simulink model "reverb"  (R2024a)
settings: Solver=VariableStepAuto  StartTime=0.0  StopTime=1  RelTol=1e-3
model workspace (MAT data in the model file):
  Sig = Simulink.Signal
  Sig.DataType = 'auto'
  Sig.Dimensions = -1
  Sig.DimensionsMode = 'auto'
  Sig.Complexity = 'auto'
  Sig.SampleTime = -1
  Sig.SamplingMode = 'auto'
undefined symbols (not defined in the file or in its folder): DELAY, DELAY_DIFF, DIFF_GAIN, GAIN, MIX
libraries: dspvision x1
settings Model: Creator=fermata  LastModifiedBy=fermata
settings SolverCC: AlgebraicLoopSolver=TrustRegion  MaxZcPerStep=1
settings DataIOCC: LimitDataPoints=on  SaveOutput=off  SignalLogging=off  SaveTime=off
settings OptimizationCC: ReuseModelBlockBuffer=off  LifeSpan=inf  SimCompilerOptimization=on
settings DebuggingCC: SingleTaskRateTransMsg=error  UnconnectedInputMsg=warning  UnconnectedOutputMsg=warning  UnconnectedLineMsg=warning  AllowSymbolicDim=off  SFUnexpectedBacktrackingDiag=warning  SFNoUnconditionalDefaultTransitionDiag=warning  SFExecutionAtInitializationDiag=none  ArithmeticOperatorsInVariantConditions=warning
settings ModelReferenceCC: EnableRefExpFcnMdlSchedulingChecks=on
settings SFSimCC: SimUseLocalCustomCode=off  CustomCodeUndefinedFunction=UseInterfaceOnly
settings RTWCC: RTWUseLocalCustomCode=off  GPUComputeCapability=3.5  DLArmComputeVersion=19.05
settings CodeAppCC: StateflowObjectComments=on
settings GRTTargetCC: TargetLangStandard=C89/C90 (ANSI)
settings ConfigComp: CovMetricSettings=dw  CovSaveCumulativeToWorkspaceVar=on  CovSaveSingleToWorkspaceVar=on  CovExternalEMLEnable=off  CovSFcnEnable=off

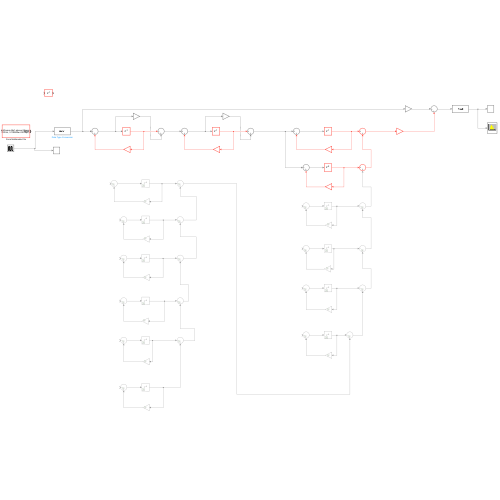
[thumbnail: Simulink's stored preview of the top-level diagram]
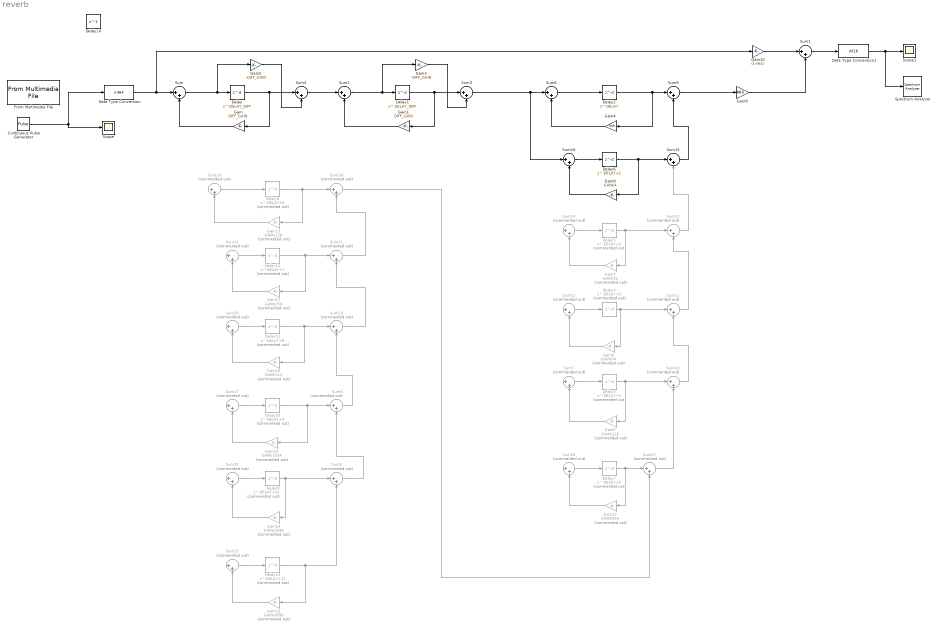
== system reverb ==
  Continuous Pulse Generator : DiscretePulseGenerator  PulseType=Time based  Amplitude=1024  Period=1
  Data Type Conversion : DataTypeConversion  OutDataTypeStr=int64  SaturateOnIntegerOverflow=off  RndMeth=Floor
  Data Type Conversion1 : DataTypeConversion  OutDataTypeStr=int16  RndMeth=Floor
  Delay : Delay  DelayLength=DELAY_DIFF  DelayLengthUpperLimit=1024  InitialCondition=0  UseCircularBuffer=on
  Delay1 : Delay  DelayLength=DELAY_DIFF  DelayLengthUpperLimit=1024  InitialCondition=0  UseCircularBuffer=on
  Delay10 : Delay  Commented=on  DelayLength=DELAY+9  DelayLengthUpperLimit=1024  InitialCondition=0  UseCircularBuffer=on
  Delay11 : Delay  Commented=on  DelayLength=DELAY+8  DelayLengthUpperLimit=1024  InitialCondition=0  UseCircularBuffer=on
  Delay12 : Delay  Commented=on  DelayLength=DELAY+7  DelayLengthUpperLimit=1024  InitialCondition=0  UseCircularBuffer=on
  Delay13 : Delay  Commented=on  DelayLength=DELAY+11  DelayLengthUpperLimit=1024  InitialCondition=0  UseCircularBuffer=on
  Delay14 : Delay  DelayLength=1  InitialCondition=0
  Delay2 : Delay  DelayLength=DELAY  DelayLengthUpperLimit=1024  InitialCondition=0  UseCircularBuffer=on
  Delay3 : Delay  Commented=on  DelayLength=DELAY+4  DelayLengthUpperLimit=1024  InitialCondition=0  UseCircularBuffer=on
  Delay4 : Delay  Commented=on  DelayLength=DELAY+3  DelayLengthUpperLimit=1024  InitialCondition=0  UseCircularBuffer=on
  Delay5 : Delay  Commented=on  DelayLength=DELAY+2  DelayLengthUpperLimit=1024  InitialCondition=0  UseCircularBuffer=on
  Delay6 : Delay  DelayLength=DELAY+1  DelayLengthUpperLimit=1024  InitialCondition=0  UseCircularBuffer=on
  Delay7 : Delay  Commented=on  DelayLength=DELAY+5  DelayLengthUpperLimit=1024  InitialCondition=0  UseCircularBuffer=on
  Delay8 : Delay  Commented=on  DelayLength=DELAY+6  DelayLengthUpperLimit=1024  InitialCondition=0  UseCircularBuffer=on
  Delay9 : Delay  Commented=on  DelayLength=DELAY+10  DelayLengthUpperLimit=1024  InitialCondition=0  UseCircularBuffer=on
  From Multimedia File : dspvision/From Multimedia File  inputFilename=/home/fermata/Development/Software/MATLAB/R2024a/toolbox/audio/samples/FunkyDrums-44p1-stereo-25secs.mp3  readRange=[1 Inf]  loop=on  numPlays=1  outputStreams=Audio only  videoDataType=single  audioDataType=int16  inheritSampleTime=on  userDefinedSampleTime=1/30  noAudioOutput=off  isIntensityVideo=off  fourcc=RGB  colorVideoFormat=One multidimensional signal  outputEOF=off  dataOrg=Column-major  audioFrameSize=1024  computeAudioFrameSize=off  outSamplingMode=Sample based
      settings: LibrarySourceBlock=dspsrcs4/From Multimedia File
  Gain : Gain  Gain=DIFF_GAIN  SaturateOnIntegerOverflow=on  OutDataTypeStr=Inherit: Same as input
  Gain1 : Gain  Gain=DIFF_GAIN  SaturateOnIntegerOverflow=on  OutDataTypeStr=Inherit: Same as input
  Gain10 : Gain  Gain=(1-MIX)
  Gain11 : Gain  Commented=on  Gain=GAIN/256  SaturateOnIntegerOverflow=on  OutDataTypeStr=Inherit: Same as input
  Gain12 : Gain  Commented=on  Gain=GAIN/4096  SaturateOnIntegerOverflow=on  OutDataTypeStr=Inherit: Same as input
  Gain13 : Gain  Commented=on  Gain=GAIN/128  SaturateOnIntegerOverflow=on  OutDataTypeStr=Inherit: Same as input
  Gain14 : Gain  Commented=on  Gain=GAIN/2048  SaturateOnIntegerOverflow=on  OutDataTypeStr=Inherit: Same as input
  Gain15 : Gain  Commented=on  Gain=GAIN/1024  SaturateOnIntegerOverflow=on  OutDataTypeStr=Inherit: Same as input
  Gain16 : Gain  Commented=on  Gain=GAIN/512  SaturateOnIntegerOverflow=on  OutDataTypeStr=Inherit: Same as input
  Gain17 : Gain  Commented=on  Gain=GAIN/256  SaturateOnIntegerOverflow=on  OutDataTypeStr=Inherit: Same as input
  Gain2 : Gain  Gain=-DIFF_GAIN  SaturateOnIntegerOverflow=on  OutDataTypeStr=Inherit: Same as input
  Gain3 : Gain  Gain=-DIFF_GAIN  SaturateOnIntegerOverflow=on  OutDataTypeStr=Inherit: Same as input
  Gain4 : Gain  Gain=GAIN  SaturateOnIntegerOverflow=on  OutDataTypeStr=Inherit: Same as input
  Gain5 : Gain  Commented=on  Gain=GAIN/128  SaturateOnIntegerOverflow=on  OutDataTypeStr=Inherit: Same as input
  Gain6 : Gain  Commented=on  Gain=GAIN/64  SaturateOnIntegerOverflow=on  OutDataTypeStr=Inherit: Same as input
  Gain7 : Gain  Commented=on  Gain=GAIN/32  SaturateOnIntegerOverflow=on  OutDataTypeStr=Inherit: Same as input
  Gain8 : Gain  Gain=GAIN/4  SaturateOnIntegerOverflow=on  OutDataTypeStr=Inherit: Same as input
  Gain9 : Gain  Gain=MIX  OutDataTypeStr=Inherit: Same as input
  Scope : Scope
  Scope1 : Scope
  Spectrum Analyzer : SpectrumAnalyzer  WindowPosition=[204.000000,780.000000,5.000000,5.000000,]  Visible=on  ScopeFrameLocation=window  SampleRateSource=Property  SampleRate=44.1e3  PlotAsTwoSidedSpectrum=off  FrequencyScale=Log  FrequencySpan=Start and stop frequencies  StartFrequency=20  StopFrequency=20e3  YLimits=[-1,1]
  Sum{,1..4,6,9,15..16} (9 alike) : Sum  Inputs=|++  SaturateOnIntegerOverflow=on
  Sum{5,7..8,10..14,17..27} (19 alike) : Sum  Commented=on  Inputs=|++  SaturateOnIntegerOverflow=on
  wires:
  Delay/1 -> Sum4/1, Gain/1
  Gain10/1 -> Sum1/1
  Sum/1 -> Gain2/1, Delay/1
  Sum1/1 -> Data Type Conversion1/1
  Gain2/1 -> Sum4/2
  Gain/1 -> Sum/2
  Gain9/1 -> Sum1/2
  Data Type Conversion/1 -> Sum/1, Gain10/1
  Gain4/1 -> Sum6/2
  Delay2/1 -> Sum9/1, Gain4/1
  Sum6/1 -> Delay2/1
  Sum7/1 -> Delay3/1
  Delay3/1 -> Sum10/1, Gain5/1
  Sum9/1 -> Gain9/1
  Gain5/1 -> Sum7/2
  Delay4/1 -> Sum11/1, Gain6/1
  Gain6/1 -> Sum12/2
  Sum12/1 -> Delay4/1
  Delay5/1 -> Sum13/1, Gain7/1
  Gain7/1 -> Sum14/2
  Sum14/1 -> Delay5/1
  Delay6/1 -> Sum15/1, Gain8/1
  Gain8/1 -> Sum16/2
  Sum16/1 -> Delay6/1
  Gain11/1 -> Sum18/2
  Sum18/1 -> Delay7/1
  Delay7/1 -> Sum27/1, Gain11/1
  Sum10/1 -> Sum11/2
  Sum11/1 -> Sum13/2
  Sum13/1 -> Sum15/2
  Sum15/1 -> Sum9/2
  Gain1/1 -> Sum2/2
  Gain3/1 -> Sum3/2
  Sum2/1 -> Gain3/1, Delay1/1
  Delay1/1 -> Sum3/1, Gain1/1
  Delay11/1 -> Sum19/1, Gain16/1
  Sum23/1 -> Delay13/1
  Gain13/1 -> Sum24/2
  Sum24/1 -> Delay8/1
  Delay10/1 -> Sum8/1, Gain15/1
  Gain15/1 -> Sum17/2
  Gain14/1 -> Sum25/2
  Delay13/1 -> Sum5/2, Gain12/1
  Sum20/1 -> Delay11/1
  Sum22/1 -> Delay12/1
  Sum19/1 -> Sum21/2
  Gain12/1 -> Sum23/2
  Sum5/1 -> Sum8/2
  Delay8/1 -> Sum26/1, Gain13/1
  Delay9/1 -> Sum5/1, Gain14/1
  Gain17/1 -> Sum22/2
  Sum21/1 -> Sum26/2
  Delay12/1 -> Sum21/1, Gain17/1
  Gain16/1 -> Sum20/2
  Sum4/1 -> Sum2/1
  Sum8/1 -> Sum19/2
  Sum25/1 -> Delay9/1
  Sum17/1 -> Delay10/1
  Sum27/1 -> Sum10/2
  Sum26/1 -> Sum27/2
  Continuous Pulse Generator/1 -> Scope/1, Data Type Conversion/1
  Sum3/1 -> Sum16/1, Sum6/1
  Data Type Conversion1/1 -> Scope1/1, Spectrum Analyzer/1
